simulink model "velo_id_gain"  (R2015a)
settings: Solver=ode3  StartTime=0.0  StopTime=5.0  RelTol=1e-3
values from neighbouring files (symbols this model uses):
  u_ini = 1.5    [velo_id_gain_mat.m]
  u_ref = u_ref_list(i)    [velo_id_gain_mat.m]
libraries: arduinolib x2
settings Model: SimulationMode=external  ExtModeTrigDuration=2  Creator=shohei  LastModifiedBy=shohei
settings OptimizationCC: OptimizeModelRefInitCode=on  LifeSpan=1
settings DebuggingCC: UnderspecifiedInitializationDetection=Classic  MergeDetectMultiDrivingBlocksExec=none
settings HardwareCC: ProdBitPerInt=16  ProdBitPerPointer=8  ProdIntDivRoundTo=Zero  ProdEndianess=LittleEndian  ProdWordSize=8  ProdHWDeviceType=Atmel->AVR
settings RTWCC: SystemTargetFile=realtime.tlc  GenerateMakefile=off  TemplateMakefile=realtime.tmf  Description=Run on Target Hardware  RTWVerbose=off
settings ERTTargetCC: CombineOutputUpdateFcns=off  ExtMode=on  ExtModeTransport=3  ExtModeMexFile=ext_serial_win32_comm_rtt  ExtModeMexArgs=0 '/dev/cu.usbmodem1421' 115200 5  ERTSrcFileBannerTemplate=realtime_code_template.cgt  ERTHdrFileBannerTemplate=realtime_code_template.cgt  ERTDataSrcFileTemplate=realtime_code_template.cgt  ERTDataHdrFileTemplate=realtime_code_template.cgt  ERTCustomFileTemplate=realtime_file_process.tlc

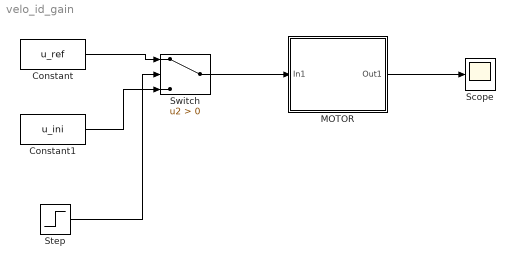
== system velo_id_gain ==
  Constant : Constant  Value=u_ref
  Constant1 : Constant  Value=u_ini
  "MOTOR " : Subsystem
  Scope : Scope
      settings: SaveName=yout
  Step : Step  SampleTime=0
  Switch : Switch  Criteria=u2 > Threshold
  wires:
  Constant1/1 -> Switch/3
  "MOTOR "/1(Out1) -> Scope/1
  Constant/1 -> Switch/1
  Step/1 -> Switch/2
  Switch/1 -> "MOTOR "/1(In1)

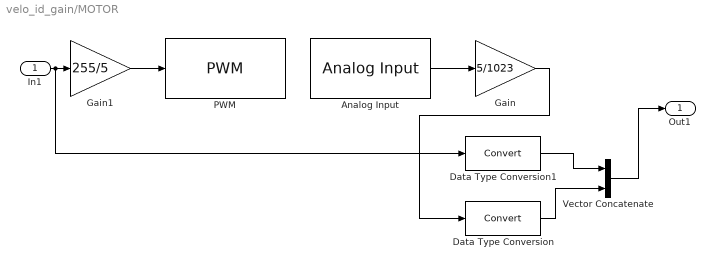
== system velo_id_gain/MOTOR  ==
  In1 : Inport
  Analog Input : arduinolib/Analog Input  pinNumber=5  sampleTime=0.01  blockPlatform=arduino
  Data Type Conversion : DataTypeConversion
  Data Type Conversion1 : DataTypeConversion
  Gain : Gain  Gain=5/1023
  Gain1 : Gain  Gain=255/5
  PWM : arduinolib/PWM  pinNumber=9  blockPlatform=arduino
  Vector Concatenate : Concatenate
  Out1 : Outport
  wires:
  In1/1 -> Data Type Conversion1/1, Gain1/1
  Analog Input/1 -> Gain/1
  Gain1/1 -> PWM/1
  Gain/1 -> Data Type Conversion/1
  Data Type Conversion1/1 -> Vector Concatenate/1
  Data Type Conversion/1 -> Vector Concatenate/2
  Vector Concatenate/1 -> Out1/1
